simulink model "a27_sim"  (R2014a)
settings: Solver=FixedStepDiscrete  StartTime=0.0  StopTime=10.0  FixedStep=0.1  RelTol=1e-3
settings Model: Creator=s65556  LastModifiedBy=s65556

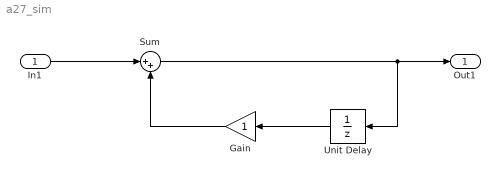
== system a27_sim ==
  In1 : Inport
  Gain : Gain
  Sum : Sum  Inputs=|++
  Unit Delay : UnitDelay  SampleTime=-1
  Out1 : Outport
  wires:
  In1/1 -> Sum/1
  Gain/1 -> Sum/2
  Unit Delay/1 -> Gain/1
  Sum/1 -> Unit Delay/1, Out1/1
